simulink model "W2_Problem_3"  (R2020a)
settings: Solver=ode45  StartTime=0.0  StopTime=120  RelTol=1e-3
values from neighbouring files (symbols this model uses):
  b = 50.0    [W2_P3_DD.sldd]
  Kd = 1.0    [W2_P3_DD.sldd]
  Ki = 1.0    [W2_P3_DD.sldd]
  Kp = 1.0    [W2_P3_DD.sldd]
  m = 1000.0    [W2_P3_DD.sldd]
settings Model: DataDictionary=W2_P3_DD.sldd  Creator=user  LastModifiedBy=user

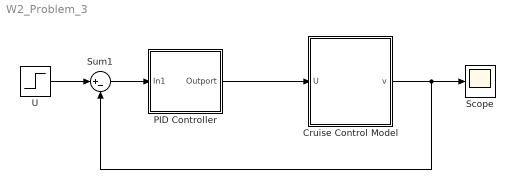
== system W2_Problem_3 ==
  Cruise Control Model : Subsystem
  PID Controller : Subsystem
  Scope : Scope
  Sum1 : Sum  Inputs=|+-
  U : Step  After=500  SampleTime=0
  wires:
  PID Controller/1(Outport) -> Cruise Control Model/1(U)
  Cruise Control Model/1(v) -> Sum1/2, Scope/1
  Sum1/1 -> PID Controller/1(In1)
  U/1 -> Sum1/1

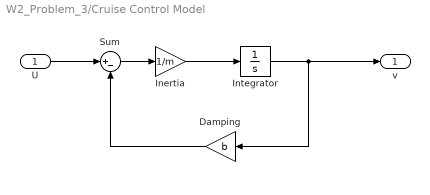
== system W2_Problem_3/Cruise Control Model ==
  U : Inport
  Damping : Gain  Gain=b
  Inertia : Gain  Gain=1/m
  Integrator : Integrator
  Sum : Sum  Inputs=|+-
  v : Outport
  wires:
  Integrator/1 -> v/1, Damping/1
  Inertia/1 -> Integrator/1
  Damping/1 -> Sum/2
  U/1 -> Sum/1
  Sum/1 -> Inertia/1

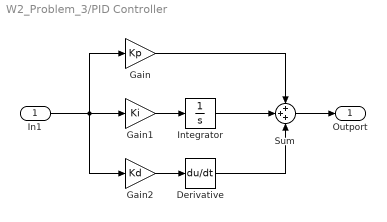
== system W2_Problem_3/PID Controller ==
  In1 : Inport
  Derivative : Derivative
  Gain : Gain  Gain=Kp
  Gain1 : Gain  Gain=Ki
  Gain2 : Gain  Gain=Kd
  Integrator : Integrator
  Sum : Sum  Inputs=+++
  Outport : Outport
  wires:
  Integrator/1 -> Sum/2
  Gain2/1 -> Derivative/1
  Derivative/1 -> Sum/3
  Sum/1 -> Outport/1
  Gain/1 -> Sum/1
  Gain1/1 -> Integrator/1
  In1/1 -> Gain2/1, Gain/1, Gain1/1
